simulink model "Aearial_Inspection_UAV_Simulation"  (R2023a)
settings: Solver=daessc  StartTime=0.0  StopTime=tf  MaxStep=0.1  MinStep=1e-30  RelTol=1e-4
values from neighbouring files (symbols this model uses):
  arm_start = 0    [InitScript.m]
  X = T*[x0;y0]    [line2circle.m]
undefined symbols (not defined in the file or in its folder): arm_end, DiscIntNeverNeededParam, F, is_gust_active, Light, MIL, Mode, Motor_data, params, Robotic_Arm_ASM_DataFile, Sensor_err, servo_specs, simple_env, stepper, Tm, wind_speed, xStack1, xStack2, Y, Z
libraries: sm_lib x399, nesl_utility x78, simulink x25, dspsrcs4 x16, simulink_extras x8, sharedtransform x7, aerolibwind2 x2, sharedutil x1
(part 1 of 12)
settings Model: Creator=mojta  LastModifiedBy=mojtaba
settings SolverCC: ZeroCrossControl=DisableAll
settings DebuggingCC: MaxConsecutiveZCsMsg=none  MaskedZcDiagnostic=none  IgnoredZcDiagnostic=none  UnconnectedInputMsg=warning  UnconnectedOutputMsg=warning  UnconnectedLineMsg=warning
settings ModelReferenceCC: EnableRefExpFcnMdlSchedulingChecks=on
settings RTWCC: DLArmComputeVersion=19.05
settings DiagnosticsConfigSet: SimMechanicsInvalidVisualProperty=none  SimMechanicsCrossSectionNullEdge=none  SimMechanicsRigidlyBoundBlock=none  SimMechanicsUnsatisfiedHighPriorityTargets=none

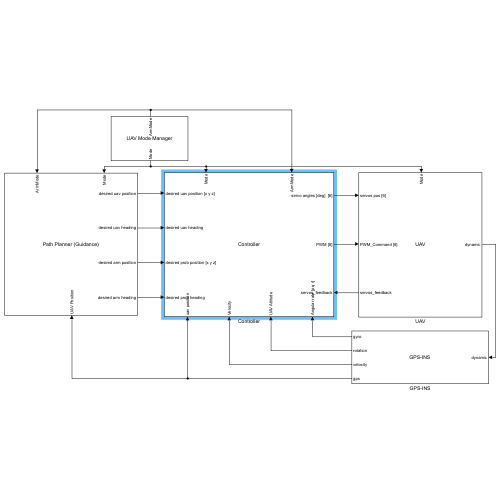
[thumbnail: Simulink's stored preview of the top-level diagram]
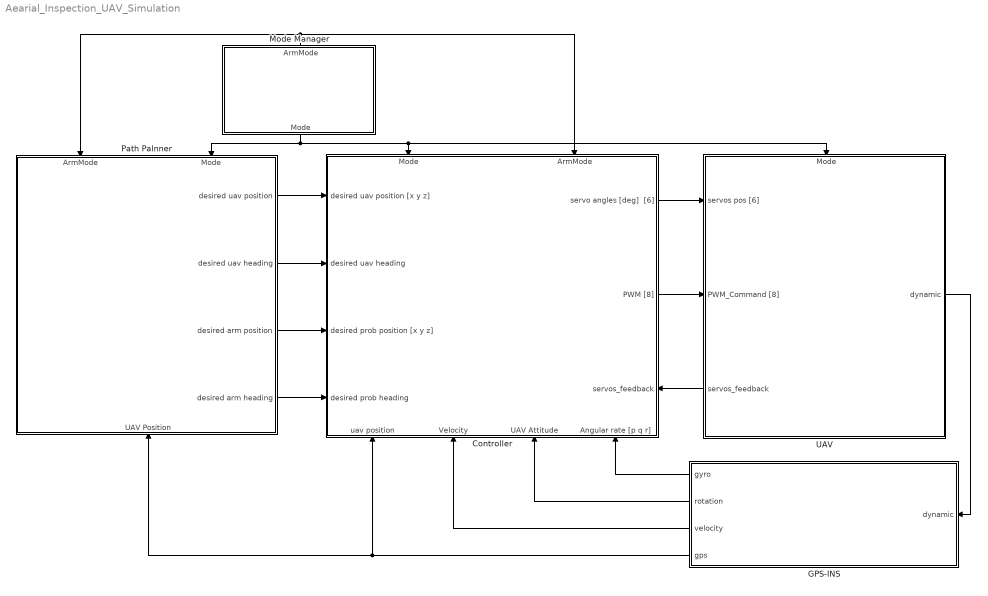
== system Aearial_Inspection_UAV_Simulation ==
  Controller : Subsystem
      settings: PortSchema="{\"entries\":[{\"content\":{\"sides\":[{\"content\":{\"connectorIds\":[\"In1\",\"In2\",\"In3\",\"In4\"]},\"type\":\"ConnectorPlacement.EquallySpacedRectSide\",\"uuid\":\"8cd7dc0d-1ffe-404b-8963-ef178fa92e53\"},{\"content\":{\"connectorIds\":[\"Out1\",\"Out2\",\"In11\"],\"side\":\"RIGHT\"},\"type\":\"ConnectorPlacement.EquallySpacedRectSide\",\"uuid\":\"919e0896-43af-402c-8143-9d4be52422e2\"},{\"content\":{\"connectorIds\":[\"In5\",\"In6\"],\"side\":\"TOP\"},\"type\":\"ConnectorPlacement.EquallySpacedRectSide\",\"uuid\":\"8ba6d734-f5ce-449a-9fca-978ebb325dd5\"},{\"content\":{\"connectorIds\":[\"In7\",\"In8\",\"In9\",\"In10\"],\"side\":\"BOTTOM\"},\"type\":\"ConnectorPlacement.EquallySpacedRectSide\",\"uuid\":\"341a769c-6dc0-48cd-a2a1-c1e2b0790a55\"}]},\"type\":\"ConnectorPlacement.EquallySpacedConnector\",\"uuid\":\"44d8020b-63e9-4f33-a120-ebcdce44349b\"}],\"packageUris\":[\"http://schema.mathworks.com/mf0/Connector/R2020b\"],\"version\":\"1.0\"}"
      mask Display: disp("Controller")
  GPS-INS : Subsystem
      mask Display: disp("GPS-INS")
  Mode Manager : Subsystem
      settings: PortSchema="{\"entries\":[{\"content\":{\"sides\":[{\"content\":{\"connectorIds\":[]},\"type\":\"ConnectorPlacement.EquallySpacedRectSide\",\"uuid\":\"ec3a6880-5567-4991-bb36-5b29953083f3\"},{\"content\":{\"connectorIds\":[],\"side\":\"RIGHT\"},\"type\":\"ConnectorPlacement.EquallySpacedRectSide\",\"uuid\":\"14318ee4-cc5e-4862-93f9-df06206ade9b\"},{\"content\":{\"connectorIds\":[\"Out2\"],\"side\":\"TOP\"},\"type\":\"ConnectorPlacement.EquallySpacedRectSide\",\"uuid\":\"762206d4-62cf-4133-8d53-9df821ce7e2e\"},{\"content\":{\"connectorIds\":[\"Out1\"],\"side\":\"BOTTOM\"},\"type\":\"ConnectorPlacement.EquallySpacedRectSide\",\"uuid\":\"6ead698c-d941-4f89-8f8b-414954de099a\"}]},\"type\":\"ConnectorPlacement.EquallySpacedConnector\",\"uuid\":\"33a2902f-a2fb-4f7e-8949-163cea2e732b\"}],\"packageUris\":[\"http://schema.mathworks.com/mf0/Connector/R2020b\"],\"version\":\"1.0\"}"
      mask Display: disp("UAV Mode Manager")
  Path Palnner : Subsystem
      settings: PortSchema="{\"entries\":[{\"content\":{\"sides\":[{\"content\":{\"connectorIds\":[]},\"type\":\"ConnectorPlacement.EquallySpacedRectSide\",\"uuid\":\"cb7ac4db-aadb-4fa9-9def-50252c1063a6\"},{\"content\":{\"connectorIds\":[\"Out1\",\"Out2\",\"Out3\",\"Out4\"],\"side\":\"RIGHT\"},\"type\":\"ConnectorPlacement.EquallySpacedRectSide\",\"uuid\":\"a421e774-a0ba-45ee-9144-209b429c5514\"},{\"content\":{\"connectorIds\":[\"In1\",\"In2\"],\"side\":\"TOP\"},\"type\":\"ConnectorPlacement.EquallySpacedRectSide\",\"uuid\":\"c25a837e-9178-40bf-ab38-1ae27b57d077\"},{\"content\":{\"connectorIds\":[\"In3\"],\"side\":\"BOTTOM\"},\"type\":\"ConnectorPlacement.EquallySpacedRectSide\",\"uuid\":\"24b9e0e9-1a2f-43ee-9fbc-f01c4afdd7a1\"}]},\"type\":\"ConnectorPlacement.EquallySpacedConnector\",\"uuid\":\"84baf3da-c25a-43bc-ab40-c057e0230948\"}],\"packageUris\":[\"http://schema.mathworks.com/mf0/Connector/R2020b\"],\"version\":\"1.0\"}"
      mask Display: disp("Path Planner (Guidance)")
  UAV : Subsystem
      mask init:
      | smiData = Aerial_Inspection_Octa_Rotor_DataFile();
      settings: PortSchema="{\"entries\":[{\"content\":{\"sides\":[{\"content\":{\"connectorIds\":[\"In1\",\"In2\",\"Out2\"]},\"type\":\"ConnectorPlacement.EquallySpacedRectSide\",\"uuid\":\"34cc31d8-8814-4b19-86b3-8c8699fa0f58\"},{\"content\":{\"connectorIds\":[\"Out1\"],\"side\":\"RIGHT\"},\"type\":\"ConnectorPlacement.EquallySpacedRectSide\",\"uuid\":\"29abd3e3-b5bd-4578-8682-c2c7537bb156\"},{\"content\":{\"connectorIds\":[\"In3\"],\"side\":\"TOP\"},\"type\":\"ConnectorPlacement.EquallySpacedRectSide\",\"uuid\":\"5d6ec585-4a55-4272-9af8-d672968573e8\"}]},\"type\":\"ConnectorPlacement.EquallySpacedConnector\",\"uuid\":\"91ac0284-653c-4c8b-a3f9-a6bca447147a\"}],\"packageUris\":[\"http://schema.mathworks.com/mf0/Connector/R2020b\"],\"version\":\"1.0\"}"
      mask Display: disp("UAV")
  wires:
  Mode Manager/1(Mode) -> Path Palnner/2(Mode), UAV/3(Mode), Controller/5(Mode)
  Path Palnner/1(desired uav position) -> Controller/1(desired uav position [x y z])
  Path Palnner/2(desired uav heading) -> Controller/2(desired uav heading)
  Path Palnner/3(desired arm position) -> Controller/3(desired prob position [x y z])
  Path Palnner/4(desired arm heading) -> Controller/4(desired prob heading)
  UAV/1(dynamic) -> GPS-INS/1(dynamic)
  GPS-INS/4(gps) -> Path Palnner/3(UAV Position), Controller/7(uav position)
  GPS-INS/3(velocity) -> Controller/8(Velocity)
  GPS-INS/2(rotation) -> Controller/9(UAV Attitude)
  GPS-INS/1("gyro ") -> Controller/10(Angular rate [p q r])
  Controller/1(servo angles [deg]  [6]) -> UAV/1(servos pos [6])
  Controller/2(PWM [8]) -> UAV/2(PWM_Command [8])
  Mode Manager/2(ArmMode) -> Path Palnner/1(ArmMode), Controller/6(ArmMode)
  UAV/2(servos_feedback) -> Controller/11(servos_feedback)

== system Aearial_Inspection_UAV_Simulation/Controller ==
  desired uav position [x y z] : Inport
  desired uav heading : Inport  Port=2
  desired prob position [x y z] : Inport  Port=3
  desired prob heading : Inport  Port=4
  Mode : Inport  Port=5
  ArmMode : Inport  Port=6
  uav position : Inport  Port=7
  Velocity : Inport  Port=8
  UAV Attitude : Inport  Port=9
  Angular rate [p q r] : Inport  Port=10
  servos_feedback : Inport  Port=11
  Arm Controller : Subsystem
      mask Display: disp("Arm Controller")
  Mixer : Subsystem
      mask init:
      | temp = Excel_Data;
      | 
      | Kt  = temp.K_T(1);
      | Km = temp.K_M(1);
      | r     = temp.d_motor;
      | 
      | K_ESC = zeros(8);
      | 
      | K_ESC(1,:)    = -Kt;
      | K_ESC(5:8,:) = [eye(4), -eye(4)];
      | 
      | for i=1:8
      | K_ESC(2,i) = -Kt*r(i,2);
      | K_ESC(3,i) = Kt*r(i,1);
      | K_ESC(4,i) = (-1)^(i)*Km;
      | end
      | 
      | inv_K_ESC = K_ESC^-1;
      | 
      | 
      | th = [0 0.5 0.55 0.6 0.65 0.75 0.85 1.]';
      | w = [0
      |     3703
      | 4005
      | 4289
      | 4575
      | 5091
      | 5635
      | 6374];
      | 
      | order = 3;
      | n = length(th);
      | A = zeros(n, order-1);
      | for i = 1 : n
      |     for j = 1:order
      |         A(i,j) = w(i)^j;
      |     end
      | end
      | 
      | a = (A'*A)^-1*A'*th;
      mask Display: disp("Mixer")
  To Workspace : ToWorkspace  VariableName=des_prob_pos  SaveFormat=Timeseries  SampleTime=-1
  UAV Controller : Subsystem
      mask init:
      | wc_Alt = 20;
      | 
      | wq = 200;
      | wp = wq;
      | wr = 50;
      | 
      | wc_x = 2;
      mask Display: disp("UAV Controller")
  servo angles [deg]  [6] : Outport
  PWM [8] : Outport  Port=2
  wires:
  UAV Controller/1(Controller Output [4]) -> Mixer/1(Controller output [4])
  desired prob position [x y z]/1 -> Arm Controller/1(desired prob pos [x,y,z]), To Workspace/1
  desired prob heading/1 -> Arm Controller/2(desired prob orientation)
  Mixer/1(PWM [8*1]) -> PWM [8]/1
  Arm Controller/1(servos pos [6]) -> servo angles [deg]  [6]/1
  desired uav position [x y z]/1 -> UAV Controller/1("desired position [xd, yd, zd]")
  desired uav heading/1 -> UAV Controller/2(desired Heading [psi_d])
  UAV Attitude/1 -> UAV Controller/5("Attitude (Euler Angles) [phi, theta, psi]"), Arm Controller/4(UAV Attitude)
  Angular rate [p q r]/1 -> UAV Controller/4(Angular Rate [p,q,r])
  uav position/1 -> UAV Controller/3(Position)
  Velocity/1 -> UAV Controller/6(Velocity)
  ArmMode/1 -> Arm Controller/5(ArmMode)
  Mode/1 -> Arm Controller/3(Mode)
  servos_feedback/1 -> Arm Controller/6(servos_feedback)

== system Aearial_Inspection_UAV_Simulation/GPS-INS ==
  dynamic : Inport
  GPS : Subsystem
  IMU : Subsystem
  Terminator : Terminator
  Terminator1 : Terminator
  Terminator2 : Terminator
  demux : Subsystem
  "gyro " : Outport
  rotation : Outport  Port=2
  velocity : Outport  Port=3
  gps : Outport  Port=4
  wires:
  dynamic/1 -> demux/1(Sensors)
  demux/5(Position) -> GPS/1(real Position data)
  IMU/1("gyro ") -> "gyro "/1
  IMU/4(rotation) -> rotation/1
  IMU/5(velocity IMU) -> velocity/1
  GPS/1("gps ") -> gps/1
  IMU/2(acc) -> Terminator/1
  IMU/3(mag) -> Terminator1/1
  GPS/2(gps velocity) -> Terminator2/1
  demux/1(Angular Velocity) -> IMU/1(real gyro data)
  demux/2(Quaternion) -> IMU/2(quaternions)
  demux/3(Acceleration) -> IMU/3(real acc data)
  demux/4(Velocity) -> IMU/4(real vel data)

== system Aearial_Inspection_UAV_Simulation/Mode Manager ==
  AND : Logic  IconShape=distinctive  AllPortsSameDT=off  OutDataTypeStr=boolean
  Cast To Double : DataTypeConversion  OutDataTypeStr=double  SaturateOnIntegerOverflow=off  RndMeth=Floor
  Clock : Clock
  Compare To Constant : simulink/Logic and Bit Operations/Compare To Constant  relop=>=  const=arm_start  OutDataTypeStr=boolean  ZeroCross=off
  Compare To Constant1 : simulink/Logic and Bit Operations/Compare To Constant  relop=<=  const=arm_end  OutDataTypeStr=boolean  ZeroCross=off
  Constant : Constant  Value=Mode
  Mode : Outport
  ArmMode : Outport  Port=2
  wires:
  Constant/1 -> Mode/1
  Cast To Double/1 -> ArmMode/1
  Clock/1 -> Compare To Constant1/1, Compare To Constant/1
  Compare To Constant/1 -> AND/1
  Compare To Constant1/1 -> AND/2
  AND/1 -> Cast To Double/1

== system Aearial_Inspection_UAV_Simulation/Path Palnner ==
  ArmMode : Inport
  Mode : Inport  Port=2
  UAV Position : Inport  Port=3
  Arm Guid : Subsystem
      mask Display: disp("Arm Planner")
  To Workspace : ToWorkspace  VariableName=des_pos  SaveFormat=Timeseries  SampleTime=-1
  To Workspace1 : ToWorkspace  VariableName=des_psi  SaveFormat=Timeseries  SampleTime=-1
  To Workspace2 : ToWorkspace  VariableName=des_arm_pos  SaveFormat=Timeseries  SampleTime=-1
  To Workspace3 : ToWorkspace  VariableName=des_arm_heading  SaveFormat=Timeseries  SampleTime=-1
  UAV_Guid : Subsystem
      mask Display: disp("UAV Guidance")
  desired uav position : Outport
  desired uav heading : Outport  Port=2
  desired arm position : Outport  Port=3
  desired arm heading : Outport  Port=4
  wires:
  Mode/1 -> Arm Guid/1(Mode), UAV_Guid/1(Mode)
  UAV Position/1 -> Arm Guid/3(uav_pos)
  UAV_Guid/1(desired_pos) -> To Workspace/1, desired uav position/1
  UAV_Guid/2(desired Heading) -> To Workspace1/1, desired uav heading/1
  Arm Guid/2(Arm Desired Orientation) -> To Workspace3/1, desired arm heading/1
  Arm Guid/1(Arm_desired_pos) -> To Workspace2/1, desired arm position/1
  ArmMode/1 -> Arm Guid/2(ArmMode)

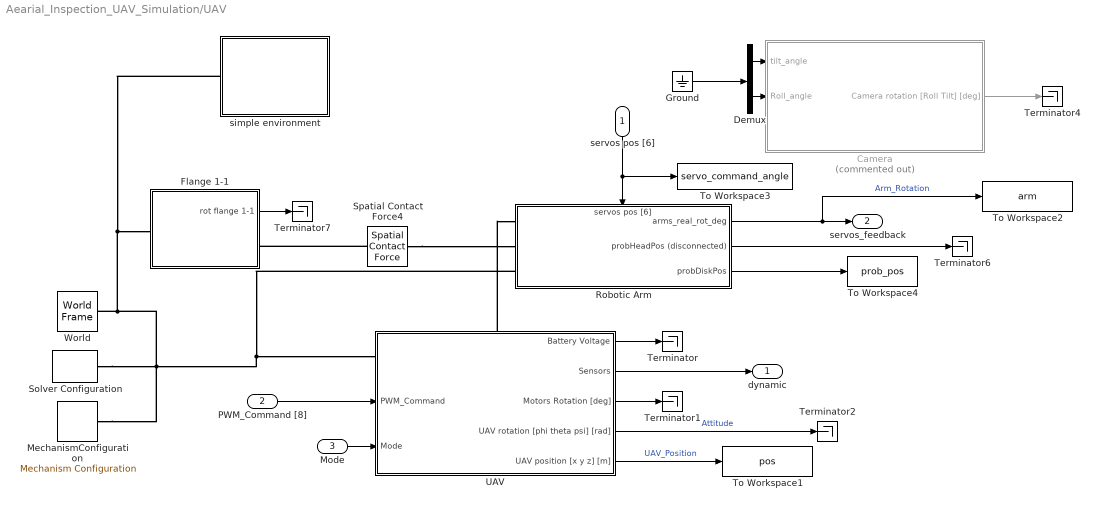
== system Aearial_Inspection_UAV_Simulation/UAV ==
  servos pos [6] : Inport  PortDimensions=6
  PWM_Command [8] : Inport  Port=2  PortDimensions=8
  Mode : Inport  Port=3
  Camera : Subsystem  Commented=on
      settings: MinAlgLoopOccurrences=on
      mask Display: image('D:\MS_Control_Project\pictures\CH3\Camera.JPG'); % Use "Edit Image" on toolstrip to change.
  Demux : Demux  Outputs=2
  Flange 1-1 : Subsystem
      mask init:
      | smiData = Flange_gate_DataFile();
      settings: MinAlgLoopOccurrences=on
  Ground : Ground
  MechanismConfiguration : sm_lib/Utilities/Mechanism Configuration  UniformGravity=Constant  GravityVector=[0 0 9.81]  GravityVectorUnits=m/s^2  LinearizationDelta=0.001  JointModeTransitionNonlinearIterations=2
  Robotic Arm : Subsystem  mask{smiData=Robotic_Arm_ASM_DataFile(), I_a0=20, I_a1=20, I_a2=20, I_w1=0.5, I_w2=0.5, I_w3=0.2, a0_maxTorque=200, a1_maxTorque=500, a2_maxTorque=200, w1_maxTorque=50, w2_maxTorque=50, w3_maxTorque=50, a0_maxVel=1, a1_maxVel=1, a2_maxVel=1, w1_maxVel=3, w2_maxVel=3, w3_maxVel=3}
      mask prompts: smiData "smData"; I_a0 "Servo a0"; I_a1 "Servo a1"; I_a2 "Servo a2"; I_w1 "Servo w1"; I_w2 "Servo w2"; I_w3 "Servo w3"; a0_maxTorque "Servo a0"; a1_maxTorque "Servo a1"; a2_maxTorque "Servo a2"; w1_maxTorque "Servo w1"; w2_maxTorque "Servo w2"; w3_maxTorque "Servo w3"; a0_maxVel "Servo a0"; a1_maxVel "Servo a1"; a2_maxVel "Servo a2"; w1_maxVel "Servo w1"; w2_maxVel "Servo w2"; w3_maxVel "Servo w3"
      mask init:
      | main
      settings: PortSchema="{\"entries\":[{\"content\":{\"sides\":[{\"content\":{\"connectorIds\":[\"LConn1\",\"LConn2\",\"LConn3\"]},\"type\":\"ConnectorPlacement.EquallySpacedRectSide\",\"uuid\":\"03f1ddf6-71cc-47f6-8398-5c3f516e61c7\"},{\"content\":{\"connectorIds\":[\"Out1\",\"Out2\",\"Out3\"],\"side\":\"RIGHT\"},\"type\":\"ConnectorPlacement.EquallySpacedRectSide\",\"uuid\":\"d8ba576a-9aaa-4705-a901-8658d79ba4ef\"},{\"content\":{\"connectorIds\":[\"In1\"],\"side\":\"TOP\"},\"type\":\"ConnectorPlacement.EquallySpacedRectSide\",\"uuid\":\"02397d5d-c4e1-4539-9121-e7da8e23bc4c\"}]},\"type\":\"ConnectorPlacement.EquallySpacedConnector\",\"uuid\":\"067dd81b-c51f-4725-9db0-fb64c43a5cf5\"}],\"packageUris\":[\"http://schema.mathworks.com/mf0/Connector/R2020b\"],\"version\":\"1.0\"}"
      mask DialogControl ParameterGroupVar Prompt: Data
      mask DialogControl ParameterGroupVar_copy Prompt: Inertia on Servos
      mask DialogControl ParameterGroupVar_copy_copy Prompt: Max Torque of Servos
      mask DialogControl ParameterGroupVar_copy_copy_copy Prompt: Max Velocity of Servos
  Solver Configuration : nesl_utility/Solver Configuration  PhysicalDomain=network_engine_domain  SubClassName=solver  LeftPortType=input  RightPortType=generic  Tones=[]  Harmonics=[]  SimulateNoise=off  Profile=off  UseLocalSampling=off  EnableSwitchedLinearOptims=on  FrequencyDomain=off  UseCCode=off  RelTol=0.001  AbsTol=1e-06  MinStep=1e-09  ToWorkspace=off  RevertToSquareIcSolve=off  NumHomotopyIterations=100  PhasorMode=off  PhasorModeNumHarmonics=1  ConsistencySolver=NEWTON_FTOL  IndexReductionMethod=DerivativeReplacement  DoDC=off  ResidualTolerance=1e-09  ConsistencyTolSource=GLOBAL  ConsistencyAbsTol=0.001  ConsistencyRelTol=0.001  ConsistencyTolFactor=0.001  UseLocalSolver=off  LocalSolverChoice=NE_BACKWARD_EULER_ADVANCER  ResolveIndetEquations=on  FunctionEvalNumThread=1  LocalSolverSampleTime=0.001  DoFixedCost=off  MaxNonlinIter=3  MaxModeIter=2  ComputeImpulses=off  ImpulseIterations=2  LinearAlgebra=auto  LinearAlgebraNumThread=0  EquationFormulation=NE_TIME_EF  DelaysMemoryBudget=1024  AutomaticFiltering=on  FilteringTimeConstant=0.001  PartitionStorageMethod=AS_NEEDED  PartitionMemoryBudget=1024  PartitionMethod=ROBUST
  Spatial Contact Force4 : sm_lib/Forces and Torques/Spatial Contact Force  SenseContactBaseRotation=off  SenseContactBaseTranslation=off  CoefficientOfDynamicFriction=0.3  CoefficientOfStaticFriction=0.5  NormalDamping=1000  NormalDampingUnits=N/(m/s)  SenseContactSignal=off  NormalStiffness=1000  NormalStiffnessUnits=N/m  FrictionalCriticalVelocity=1e-3  FrictionalCriticalVelocityUnits=m/s  ZeroCrossDetectContactStartAndEnd=off  SenseContactFollowerRotation=off  SenseContactFollowerTranslation=off  FrictionType=SmoothStickSlip  SenseFrictionalForceMagnitude=off  SenseNormalForceMagnitude=off  NormalForceType=SmoothSpringDamper  SenseNormalVelocity=off  SenseSeparationDistance=off  SenseTangentialVelocity=off  NormalTransitionRegionWidth=1e-3  NormalTransitionRegionWidthUnits=m
  Terminator{,1..2,4,6..7} (6 alike) : Terminator
  To Workspace1 : ToWorkspace  VariableName=pos  SaveFormat=Timeseries  SampleTime=-1
  To Workspace2 : ToWorkspace  VariableName=arm  SaveFormat=Timeseries  SampleTime=-1
  To Workspace3 : ToWorkspace  VariableName=servo_command_angle  SaveFormat=Timeseries  SampleTime=-1
  To Workspace4 : ToWorkspace  VariableName=prob_pos  SaveFormat=Timeseries  SampleTime=-1
  UAV : Subsystem
      settings: MinAlgLoopOccurrences=on  PortSchema="{\"entries\":[{\"content\":{\"sides\":[{\"content\":{\"connectorIds\":[\"LConn1\",\"In1\",\"In2\"]},\"type\":\"ConnectorPlacement.EquallySpacedRectSide\",\"uuid\":\"3a522cf1-0d2e-42a1-8abc-fdb0da215095\"},{\"content\":{\"connectorIds\":[\"Out1\",\"Out2\",\"Out3\",\"Out4\",\"Out5\"],\"side\":\"RIGHT\"},\"type\":\"ConnectorPlacement.EquallySpacedRectSide\",\"uuid\":\"0b06edfd-f156-4bc5-9eca-7fe97f182038\"},{\"content\":{\"connectorIds\":[\"LConn2\"],\"side\":\"TOP\"},\"type\":\"ConnectorPlacement.EquallySpacedRectSide\",\"uuid\":\"5d149f1b-6095-4c3b-bbee-46e9e9cd7497\"}]},\"type\":\"ConnectorPlacement.EquallySpacedConnector\",\"uuid\":\"072866d9-af86-4096-8e43-cca5dedb3158\"}],\"packageUris\":[\"http://schema.mathworks.com/mf0/Connector/R2020b\"],\"version\":\"1.0\"}"
      mask Display: image('D:\MS_Control_Project\pictures\CH5\UAV.JPG'); % Use "Edit Image" on toolstrip to change.
  World : sm_lib/Frames and Transforms/World Frame
  simple environment : Subsystem
  dynamic : Outport
  servos_feedback : Outport  Port=2
  wires:
  Demux/1 -> Camera/1(tilt_angle)
  PWM_Command [8]/1 -> UAV/1(PWM_Command)
  Robotic Arm/3(probDiskPos) -> To Workspace4/1
  UAV/1(Battery Voltage) -> Terminator/1
  UAV/2(Sensors) -> dynamic/1
  servos pos [6]/1 -> To Workspace3/1, Robotic Arm/1(servos pos [6])
  Flange 1-1/1(rot flange 1-1) -> Terminator7/1
  Robotic Arm/1(arms_real_rot_deg) -> servos_feedback/1, To Workspace2/1  "Arm_Rotation"
  Demux/2 -> Camera/2(Roll_angle)
  UAV/4(UAV rotation [phi theta psi] [rad]) -> Terminator2/1  "Attitude"
  Ground/1 -> Demux/1
  Camera/1(Camera rotation [Roll Tilt] [deg]) -> Terminator4/1
  UAV/3(Motors Rotation [deg]) -> Terminator1/1
  UAV/5(UAV position [x y z] [m]) -> To Workspace1/1  "UAV_Position"
  Robotic Arm/2(probHeadPos (disconnected)) -> Terminator6/1
  Mode/1 -> UAV/2(Mode)
  connections:
  MechanismConfiguration/RConn1 -- Solver Configuration/RConn1 -- simple environment/LConn1 -- Flange 1-1/LConn1 -- World/RConn1 -- Robotic Arm/LConn3 -- UAV/LConn1
  UAV/LConn2 -- Robotic Arm/LConn1
  Spatial Contact Force4/LConn1 -- Flange 1-1/RConn1
  Spatial Contact Force4/RConn1 -- Robotic Arm/LConn2

== system Aearial_Inspection_UAV_Simulation/Controller/Arm Controller ==
  desired prob pos [x,y,z] : Inport
  desired prob orientation : Inport  Port=2  PortDimensions=1
  Mode : Inport  Port=3
  UAV Attitude : Inport  Port=4  PortDimensions=3
  ArmMode : Inport  Port=5
  servos_feedback : Inport  Port=6
  Arm and Wrist Inv-kinematics : Subsystem
  Compare To Constant : simulink/Logic and Bit Operations/Compare To Constant  relop===  const=2  OutDataTypeStr=boolean
  Compare To Constant1 : simulink/Logic and Bit Operations/Compare To Constant  relop===  const=5  OutDataTypeStr=boolean
  Compare To Constant2 : simulink/Logic and Bit Operations/Compare To Constant  relop===  const=2  OutDataTypeStr=boolean
  Compare To Constant3 : simulink/Logic and Bit Operations/Compare To Constant  relop===  const=5  OutDataTypeStr=boolean
  Enabled Subsystem : Subsystem  TreatAsAtomicUnit=on
  NOT : Logic  Operator=NOT  IconShape=distinctive  AllPortsSameDT=off  OutDataTypeStr=boolean
  OR : Logic  Operator=OR  IconShape=distinctive  AllPortsSameDT=off  OutDataTypeStr=boolean
  Subsystem : Subsystem
  Sum : Sum  Inputs=++|
  Sum1 : Sum  Inputs=++|
  servos pos [6] : Outport
  wires:
  Compare To Constant1/1 -> Arm and Wrist Inv-kinematics/Enable
  Mode/1 -> Compare To Constant/1, Compare To Constant2/1, Compare To Constant3/1, Compare To Constant1/1, Arm and Wrist Inv-kinematics/1(Mode)
  Enabled Subsystem/1(Servo pos [6]) -> Sum1/1
  desired prob pos [x,y,z]/1 -> Arm and Wrist Inv-kinematics/2(desired prob pos [x,y,z])
  Compare To Constant/1 -> Enabled Subsystem/Enable
  desired prob orientation/1 -> Arm and Wrist Inv-kinematics/3(desired prob orientation)
  Arm and Wrist Inv-kinematics/1(servos pos [6]) -> Sum/2
  Sum/1 -> servos pos [6]/1
  UAV Attitude/1 -> Arm and Wrist Inv-kinematics/4(UAV Attitude)
  ArmMode/1 -> Arm and Wrist Inv-kinematics/5(ArmMode)
  servos_feedback/1 -> Arm and Wrist Inv-kinematics/6(servos_feedback)
  Compare To Constant2/1 -> OR/1
  Compare To Constant3/1 -> OR/2
  OR/1 -> NOT/1
  Sum1/1 -> Sum/1
  Subsystem/1(Out1) -> Sum1/2
  NOT/1 -> Subsystem/1(In1)

== system Aearial_Inspection_UAV_Simulation/Controller/Mixer ==
  Controller output [4] : Inport  PortDimensions=4
  Constant : Constant  Value=zeros(4,1)
  Constant1 : Constant  Value=3
  Gain : Gain  Gain=inv_K_ESC  Multiplication=Matrix(K*u)
  Gain1 : Gain  Gain=a(3)
  Gain2 : Gain  Gain=a(2)
  Gain3 : Gain  Gain=a(1)
  Mux : Mux  Inputs=2
  N 2 gr : Gain  Gain=[1000/9.81*[1 1 1] 1]
  Power : Math  Operator=square
  Power1 : Math  Operator=pow
  Saturation : Saturate  UpperLimit=(6374*2*pi/60)^2  LowerLimit=0  ZeroCross=off
  Saturation1 : Saturate  UpperLimit=1  LowerLimit=0  ZeroCross=off
  Scope : Scope
  Scope1 : Scope
  Scope2 : Scope
  Sqrt : Sqrt
  Sum : Sum  Inputs=3
  rad/s to RPM : Gain  Gain=60/2/pi
  PWM [8*1] : Outport
  wires:
  N 2 gr/1 -> Mux/1
  Saturation1/1 -> Scope/1, PWM [8*1]/1
  Gain1/1 -> Sum/1
  Gain3/1 -> Sum/3
  Controller output [4]/1 -> Scope1/1, N 2 gr/1
  Saturation/1 -> Sqrt/1
  rad/s to RPM/1 -> Scope2/1, Gain3/1, Power1/1, Power/1
  Gain2/1 -> Sum/2
  Sqrt/1 -> rad/s to RPM/1
  Power/1 -> Gain2/1
  Sum/1 -> Saturation1/1
  Constant/1 -> Mux/2
  Power1/1 -> Gain1/1
  Constant1/1 -> Power1/2
  Mux/1 -> Gain/1
  Gain/1 -> Saturation/1

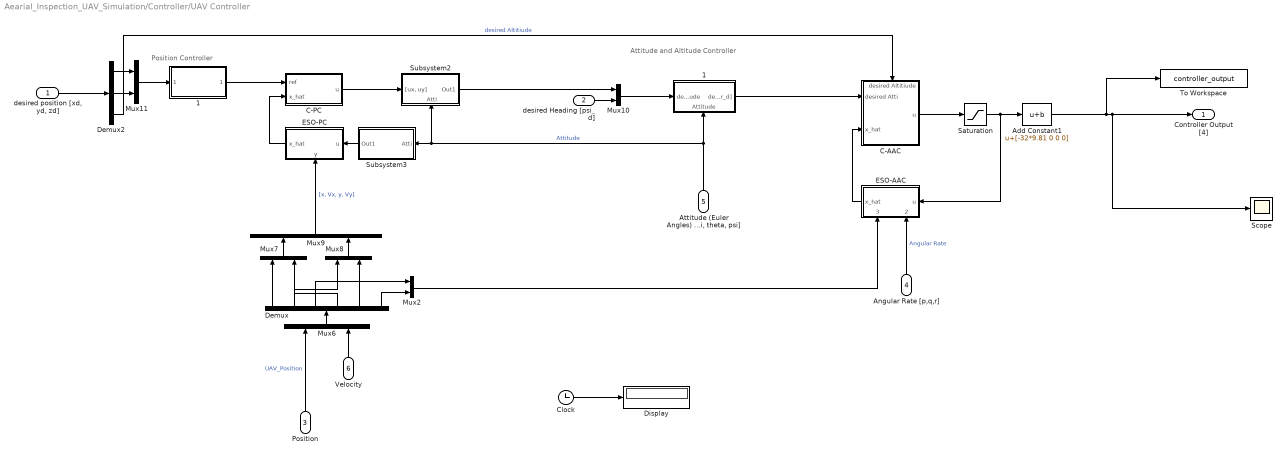
== system Aearial_Inspection_UAV_Simulation/Controller/UAV Controller ==
  note: Attitude and Altitude Controller
  note: Position Controller
  "desired position [xd, yd, zd]" : Inport  PortDimensions=3
  desired Heading [psi_d] : Inport  Port=2  PortDimensions=1
  Position : Inport  Port=3  PortDimensions=3
  Angular Rate [p,q,r] : Inport  Port=4  PortDimensions=3
  "Attitude (Euler Angles) [phi, theta, psi]" : Inport  Port=5  PortDimensions=3
  Velocity : Inport  Port=6  PortDimensions=3
  "      1" : Subsystem  mask{ff_on=0, wphi=wp/4, wpsi=wr/4}
      mask prompts: ff_on "is Feed Forward Enable"; wphi "phi and theta Channel freq"; wpsi "psi Channel freq"
      mask init:
      | K = [wphi 0 0;0 wphi 0;0 0 wpsi];
      | C = [0 ff_on      0 0      0 0
      |      0 0      0 ff_on      0 0
      |      0 0      0 0      0 ff_on];
      settings: PortSchema="{\"entries\":[{\"content\":{\"sides\":[{\"content\":{\"connectorIds\":[\"In1\"]},\"type\":\"ConnectorPlacement.EquallySpacedRectSide\",\"uuid\":\"d7bfb74f-f0ef-45e8-b402-84c976e030ff\"},{\"content\":{\"connectorIds\":[\"Out1\"],\"side\":\"RIGHT\"},\"type\":\"ConnectorPlacement.EquallySpacedRectSide\",\"uuid\":\"7a56635f-9db1-4285-a1b6-a2387fe77a8c\"},{\"content\":{\"connectorIds\":[],\"side\":\"TOP\"},\"type\":\"ConnectorPlacement.EquallySpacedRectSide\",\"uuid\":\"8927570d-ca43-4684-a275-ba6cf3010bd2\"},{\"content\":{\"connectorIds\":[\"In2\"],\"side\":\"BOTTOM\"},\"type\":\"ConnectorPlacement.EquallySpacedRectSide\",\"uuid\":\"c03033a2-2d15-4ba6-80ad-a3592136c9e5\"}]},\"type\":\"ConnectorPlacement.EquallySpacedConnector\",\"uuid\":\"5c6a6a0d-05db-4861-9314-e27434e60dad\"}],\"packageUris\":[\"http://schema.mathworks.com/mf0/Connector/R2020b\"],\"version\":\"1.0\"}"
      mask Display: disp("EU2BAR")
  "     1" : Subsystem  mask{wx=50, wy=50}
      mask init:
      | Bx = zeros(3,1);
      | Bx(end) = wx^3;
      | 
      | Ax = zeros(3);
      | Ax(1,2) = 1;
      | Ax(2,3) = 1;
      | Ax(end,:) = [-wx^3 -3*wx^2 -3*wx];
      | 
      | By = zeros(3,1);
      | By(end) = wy^3;
      | 
      | Ay = zeros(3);
      | Ay(1,2) = 1;
      | Ay(2,3) = 1;
      | Ay(end,:) = [-wy^3 -3*wy^2 -3*wy];
      mask Display: disp("TD-PC")
  Add Constant1 : Bias  Bias=[-32*9.81 0 0 0]  SaturateOnIntegerOverflow=off
  "C-AAC " : Subsystem
      settings: PortSchema="{\"entries\":[{\"content\":{\"sides\":[{\"content\":{\"connectorIds\":[\"In1\",\"In2\"]},\"type\":\"ConnectorPlacement.EquallySpacedRectSide\",\"uuid\":\"0074a7af-5369-4567-a570-5214c890c1e4\"},{\"content\":{\"connectorIds\":[\"Out1\"],\"side\":\"RIGHT\"},\"type\":\"ConnectorPlacement.EquallySpacedRectSide\",\"uuid\":\"74f23e42-f7b0-4104-8eab-960110f0734e\"},{\"content\":{\"connectorIds\":[\"In3\"],\"side\":\"TOP\"},\"type\":\"ConnectorPlacement.EquallySpacedRectSide\",\"uuid\":\"3809b58d-5d28-4fa1-bb5c-40abfdb463ef\"}]},\"type\":\"ConnectorPlacement.EquallySpacedConnector\",\"uuid\":\"2144d4c9-afd4-4ceb-a08a-cb907e035127\"}],\"packageUris\":[\"http://schema.mathworks.com/mf0/Connector/R2020b\"],\"version\":\"1.0\"}"
  C-PC : Subsystem
  Clock : Clock
  Demux : Demux  Outputs=6
  Demux2 : Demux  Outputs=3
  Display : Display
  ESO-AAC : Subsystem  mask{w_z=wc_Alt/2, w_p=wp/2, w_q=wq/2, w_r=wr/2, zeta=1}
      mask prompts: w_z "Alt Channel freq"; w_p "roll Channel freq"; w_q "pitch Channel freq"; w_r "yaw Channel freq"; zeta "damping coef"
      mask init:
      | C = [eye(5) zeros(5,4)];
      | 
      | params = Excel_Data;
      | m = params.M;
      | I = params.I;
      | 
      | Ix = I(1,1);
      | Iy = I(2,2);
      | Iz = I(3,3);
      | Ixz = I(1,3);
      | 
      | B = [0 0 0 0;1/m 0 0 0;0 Iz/(Iz*Ix-Ixz^2) 0 -Ixz/(Iz*Ix-Ixz^2);
      |      0 0 1/Iy 0;0 -Ixz/(Iz*Ix-Ixz^2) 0 Ix/(Iz*Ix-Ixz^2);zeros(4)];
      | 
      | L1 = 3*w_z;
      | L2 = 3*w_z^2;
      | L7 = m*w_z^3; 
      |  
      | L4 = 2*zeta*w_q;
      | L6 = (0.25*L4^2 + w_q^2*(1-zeta^2))/0.250549;
      | 
      | L3 = 2*zeta*w_p;
      | L5 = w_p^2*Ix;
      | 
      | L8 = 2*zeta*w_r;
      | L9 = w_r^2*Iz;
      | 
      | % syms L3 L5 L8 L9 L10 L11 a1 a2 a3 s wz wx real
      | 
      | A1 = [0 1 0 0 0;
      |     zeros(4,5)];
      | 
      | B1 = [0 0 0 0;1/m 0 0 0;zeros(3,1) I^-1];
      | A = [A1 B1
      |     zeros(4,9)];
      | 
      | 
      | L = [L1 0 0 0 0;L2 0 0 0 0;0 0 L3 0 0;0 0 0 L4 0;0 0 0 0 L8;L7 0 0 0 0;0 0 L5 0 0;
      |      0  0 0 L6 0; 0 0 0 0 L9];
      |  
      | eig(A-L*C)
      settings: PortSchema="{\"entries\":[{\"content\":{\"sides\":[{\"content\":{\"connectorIds\":[\"In1\"]},\"type\":\"ConnectorPlacement.EquallySpacedRectSide\",\"uuid\":\"d7bfb74f-f0ef-45e8-b402-84c976e030ff\"},{\"content\":{\"connectorIds\":[\"Out1\"],\"side\":\"RIGHT\"},\"type\":\"ConnectorPlacement.EquallySpacedRectSide\",\"uuid\":\"7a56635f-9db1-4285-a1b6-a2387fe77a8c\"},{\"content\":{\"connectorIds\":[],\"side\":\"TOP\"},\"type\":\"ConnectorPlacement.EquallySpacedRectSide\",\"uuid\":\"8927570d-ca43-4684-a275-ba6cf3010bd2\"},{\"content\":{\"connectorIds\":[\"In2\",\"In3\"],\"side\":\"BOTTOM\"},\"type\":\"ConnectorPlacement.EquallySpacedRectSide\",\"uuid\":\"f91df5b2-ed55-4d65-a094-b76377ad5e05\"}]},\"type\":\"ConnectorPlacement.EquallySpacedConnector\",\"uuid\":\"5c6a6a0d-05db-4861-9314-e27434e60dad\"}],\"packageUris\":[\"http://schema.mathworks.com/mf0/Connector/R2020b\"],\"version\":\"1.0\"}"
      mask Display: disp("ESO-AAC")
  ESO-PC : Subsystem  mask{w=wc_x}
      mask prompts: w "natural freq of complex pole"
      mask init:
      | L1 = 3*w;
      | L2 = 3*w^2;
      | L3 = w^3;
      | 
      | L4 = L1;
      | L5 = L2;
      | L6 = L3;
      | 
      | L = [L1 0 0 0;
      |      L2 0 0 0 
      |      0 0 L4 0
      |      0 0 L5 0
      |      L3 0 0 0
      |      0 0 L6 0];
      | 
      | A = [0 1 0 0
      |      0 0 0 0
      |      0 0 0 1
      |      0 0 0 0];
      | M = [0 0
      |     1 0
      |     0 0
      |     0 1];
      | C = [eye(4) zeros(4,2)];
      | 
      | A = [A M;zeros(2,6)];
      | 
      | B = [0 0;1 0;0 0;0 1;0 0;0 0];
      settings: PortSchema="{\"entries\":[{\"content\":{\"sides\":[{\"content\":{\"connectorIds\":[\"In1\"]},\"type\":\"ConnectorPlacement.EquallySpacedRectSide\",\"uuid\":\"d7bfb74f-f0ef-45e8-b402-84c976e030ff\"},{\"content\":{\"connectorIds\":[\"Out1\"],\"side\":\"RIGHT\"},\"type\":\"ConnectorPlacement.EquallySpacedRectSide\",\"uuid\":\"7a56635f-9db1-4285-a1b6-a2387fe77a8c\"},{\"content\":{\"connectorIds\":[],\"side\":\"TOP\"},\"type\":\"ConnectorPlacement.EquallySpacedRectSide\",\"uuid\":\"8927570d-ca43-4684-a275-ba6cf3010bd2\"},{\"content\":{\"connectorIds\":[\"In2\"],\"side\":\"BOTTOM\"},\"type\":\"ConnectorPlacement.EquallySpacedRectSide\",\"uuid\":\"2b6c045b-0b63-4552-873e-a472e925fa36\"}]},\"type\":\"ConnectorPlacement.EquallySpacedConnector\",\"uuid\":\"5c6a6a0d-05db-4861-9314-e27434e60dad\"}],\"packageUris\":[\"http://schema.mathworks.com/mf0/Connector/R2020b\"],\"version\":\"1.0\"}"
      mask Display: disp("ESO-PC")
  Mux{2,6..11} (7 alike) : Mux  Inputs=2
  Saturation : Saturate  UpperLimit=[150 100 100 1.8*4]  LowerLimit=[-150 -100 -100 -1.8*4]  ZeroCross=off
  Scope : Scope
  Subsystem2 : Subsystem
      settings: PortSchema="{\"entries\":[{\"content\":{\"sides\":[{\"content\":{\"connectorIds\":[\"In1\"]},\"type\":\"ConnectorPlacement.EquallySpacedRectSide\",\"uuid\":\"1f5be12c-0015-40b2-bce0-3a0d27346b90\"},{\"content\":{\"connectorIds\":[\"Out1\"],\"side\":\"RIGHT\"},\"type\":\"ConnectorPlacement.EquallySpacedRectSide\",\"uuid\":\"d291273e-1e98-4271-b999-541a78db916f\"},{\"content\":{\"connectorIds\":[],\"side\":\"TOP\"},\"type\":\"ConnectorPlacement.EquallySpacedRectSide\",\"uuid\":\"31981d06-c4a1-43d5-a7b9-a24549041434\"},{\"content\":{\"connectorIds\":[\"In2\"],\"side\":\"BOTTOM\"},\"type\":\"ConnectorPlacement.EquallySpacedRectSide\",\"uuid\":\"660fd505-562e-46c1-ac20-75e83f511c9b\"}]},\"type\":\"ConnectorPlacement.EquallySpacedConnector\",\"uuid\":\"1e4f524b-2827-4918-a88e-6164cba08db9\"}],\"packageUris\":[\"http://schema.mathworks.com/mf0/Connector/R2020b\"],\"version\":\"1.0\"}"
      mask Display: disp("Acc2Tilt")
  Subsystem3 : Subsystem
      mask Display: disp("Tilt2Acc")
  To Workspace : ToWorkspace  VariableName=controller_output  SaveFormat=Timeseries  SampleTime=-1
  Controller Output [4] : Outport  PortDimensions=4
  wires:
  Mux2/1 -> ESO-AAC/3("[Alt, Climb rate]")
  Angular Rate [p,q,r]/1 -> ESO-AAC/2(Angular Rate [p,q,r])  "Angular Rate"
  Demux2/3 -> "C-AAC "/3(desired Altitiude)  "desired Altitiude"
  Mux8/1 -> Mux9/2
  "     1"/1("[xd, xd_dot, xd_2dot] [yd, yd_dot, yd_2dot]") -> C-PC/1(ref)
  Mux6/1 -> Demux/1
  ESO-AAC/1(x_hat) -> "C-AAC "/2(x_hat)
  Position/1 -> Mux6/1  "UAV_Position"
  C-PC/1(u) -> Subsystem2/1("[ux, uy]")
  Add Constant1/1 -> To Workspace/1, Scope/1, Controller Output [4]/1
  Demux2/2 -> Mux11/2
  ESO-PC/1(x_hat) -> C-PC/2(x_hat)
  Subsystem2/1(Out1) -> Mux10/1
  "desired position [xd, yd, zd]"/1 -> Demux2/1
  Mux11/1 -> "     1"/1("[xd, yd]")
  Mux7/1 -> Mux9/1
  Demux2/1 -> Mux11/1
  Clock/1 -> Display/1
  Mux9/1 -> ESO-PC/2(y)  "[x, Vx, y, Vy]"
  Velocity/1 -> Mux6/2
  Demux/2 -> Mux8/1
  Subsystem3/1(Out1) -> ESO-PC/1(u)
  Saturation/1 -> Add Constant1/1, ESO-AAC/1(u)
  Demux/6 -> Mux2/2
  desired Heading [psi_d]/1 -> Mux10/2
  Demux/5 -> Mux8/2
  Mux10/1 -> "      1"/1(desired Attitude)
  "Attitude (Euler Angles) [phi, theta, psi]"/1 -> "      1"/2(Attitude), Subsystem3/1(Atti), Subsystem2/2(Atti)  "Attitude"
  "      1"/1("desired Angular rate [p_d, q_d, r_d]") -> "C-AAC "/1(desired Atti)
  "C-AAC "/1(u) -> Saturation/1
  Demux/3 -> Mux2/1
  Demux/1 -> Mux7/1
  Demux/4 -> Mux7/2

== system Aearial_Inspection_UAV_Simulation/GPS-INS/GPS ==
  real Position data : Inport  PortDimensions=3
  Gain : Gain  Commented=on  Gain=Sensor_err.gps.filt
  Integrator : Integrator  Commented=on
  Subsystem : Subsystem
  Sum : Sum  Commented=on  Inputs=+-
  Transport Delay : TransportDelay  DelayTime=0.001
  "gps " : Outport
  gps velocity : Outport  Port=2
  wires:
  Transport Delay/1 -> Subsystem/1(real Position data)
  Integrator/1 -> Sum/2
  Gain/1 -> Integrator/1, gps velocity/1
  Sum/1 -> Gain/1
  Subsystem/1(gps output) -> Sum/1, "gps "/1
  real Position data/1 -> Transport Delay/1

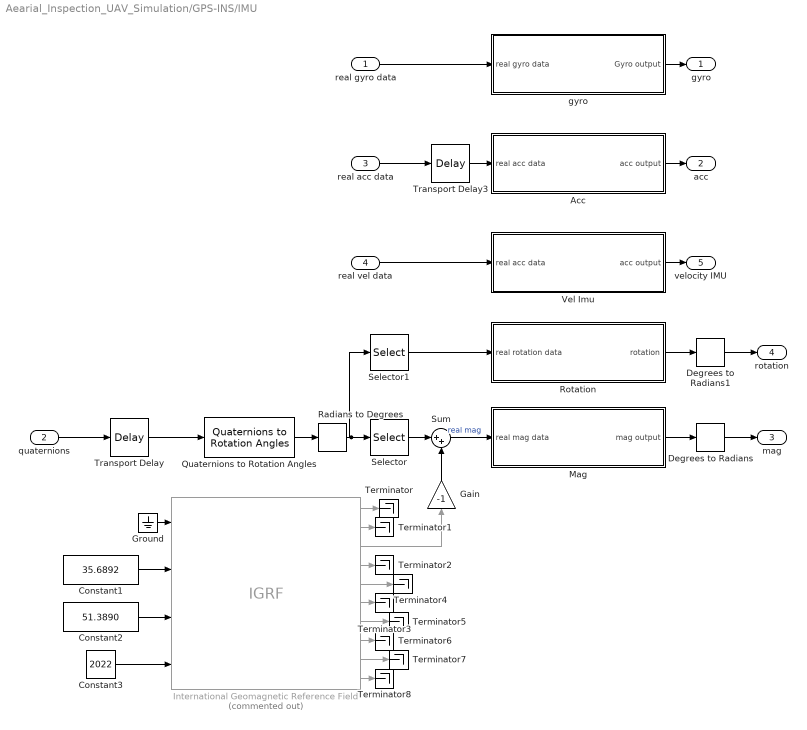
== system Aearial_Inspection_UAV_Simulation/GPS-INS/IMU ==
  real gyro data : Inport  PortDimensions=3
  quaternions : Inport  Port=2  PortDimensions=4
  real acc data : Inport  Port=3  PortDimensions=3
  real vel data : Inport  Port=4  PortDimensions=3
  Acc : Subsystem
  Constant1 : Constant  Value=35.6892
  Constant2 : Constant  Value=51.3890
  Constant3 : Constant  Value=2022
  Degrees to Radians : simulink_extras/Transformations/Degrees to Radians
  Degrees to Radians1 : simulink_extras/Transformations/Degrees to Radians
  Gain : Gain  Gain=-1
  Ground : Ground
  International Geomagnetic Reference Field : IGRF  Commented=on  month=January  day=1  year=2020
      settings: AttributesFormatString=%<generation>
  Mag : Subsystem
  Quaternions to Rotation Angles : sharedtransform/Quaternions to Rotation Angles  rotationOrder=ZYX  aMode=aMode
  Radians to Degrees : simulink_extras/Transformations/Radians to Degrees
  Rotation : Subsystem
  Selector : Selector  InputPortWidth=3  IndexOptions=Index vector (dialog)  Indices=1  OutputSizes=1
  Selector1 : Selector  InputPortWidth=3  IndexOptions=Index vector (dialog)  Indices=[3 2 1]  OutputSizes=1
  Sum : Sum  Inputs=|++
  Terminator{,1..8} (9 alike) : Terminator
  Transport Delay : TransportDelay  DelayTime=0.001  InitialOutput=[1 0 0 0]
  Transport Delay3 : TransportDelay  DelayTime=0.001
  Vel Imu : Subsystem
  gyro : Subsystem
  "gyro " : Outport
  acc : Outport  Port=2
  mag : Outport  Port=3
  rotation : Outport  Port=4
  velocity IMU : Outport  Port=5
  wires:
  Selector/1 -> Sum/1
  real acc data/1 -> Transport Delay3/1
  real vel data/1 -> Vel Imu/1(real acc data)
  International Geomagnetic Reference Field/9 -> Terminator7/1
  quaternions/1 -> Transport Delay/1
  Constant2/1 -> International Geomagnetic Reference Field/3
  International Geomagnetic Reference Field/5 -> Terminator4/1
  Ground/1 -> International Geomagnetic Reference Field/1
  Radians to Degrees/1 -> Selector1/1, Selector/1
  real gyro data/1 -> gyro/1(real gyro data)
  International Geomagnetic Reference Field/8 -> Terminator6/1
  Quaternions to Rotation Angles/1 -> Radians to Degrees/1
  Rotation/1(rotation) -> Degrees to Radians1/1
  Selector1/1 -> Rotation/1(real rotation data)
  International Geomagnetic Reference Field/7 -> Terminator5/1
  Degrees to Radians/1 -> mag/1
  Degrees to Radians1/1 -> rotation/1
  International Geomagnetic Reference Field/3 -> Gain/1
  Acc/1(acc output) -> acc/1
  International Geomagnetic Reference Field/10 -> Terminator8/1
  Constant1/1 -> International Geomagnetic Reference Field/2
  International Geomagnetic Reference Field/6 -> Terminator3/1
  Sum/1 -> Mag/1(real mag data)  "real mag"
  Vel Imu/1(acc output) -> velocity IMU/1
  International Geomagnetic Reference Field/4 -> Terminator2/1
  Mag/1(mag output) -> Degrees to Radians/1
  International Geomagnetic Reference Field/1 -> Terminator/1
  Gain/1 -> Sum/2
  International Geomagnetic Reference Field/2 -> Terminator1/1
  gyro/1(Gyro output) -> "gyro "/1
  Constant3/1 -> International Geomagnetic Reference Field/4
  Transport Delay3/1 -> Acc/1(real acc data)
  Transport Delay/1 -> Quaternions to Rotation Angles/1

== system Aearial_Inspection_UAV_Simulation/GPS-INS/demux ==
  Sensors : Inport
  Acceleration Composer : Mux  Inputs=3
  Angular Velocity Composer : Mux  Inputs=3
  Demux : Demux  Outputs=9+4+3+3
  Position Composer : Mux  Inputs=3
  Quaternion Composer : Mux
  Terminator : Terminator
  Terminator1 : Terminator
  Terminator2 : Terminator
  Velocity Composer : Mux  Inputs=3
  Angular Velocity : Outport
  Quaternion : Outport  Port=2
  Acceleration : Outport  Port=3
  Velocity : Outport  Port=4
  Position : Outport  Port=5
  wires:
  Demux/13 -> Quaternion Composer/4
  Demux/3 -> Acceleration Composer/1
  Demux/14 -> Angular Velocity Composer/1
  Demux/5 -> Velocity Composer/2
  Demux/6 -> Acceleration Composer/2
  Demux/2 -> Velocity Composer/1
  Demux/16 -> Angular Velocity Composer/3
  Demux/9 -> Acceleration Composer/3
  Demux/4 -> Position Composer/2
  Demux/1 -> Position Composer/1
  Demux/18 -> Terminator1/1
  Demux/7 -> Position Composer/3
  Demux/15 -> Angular Velocity Composer/2
  Quaternion Composer/1 -> Quaternion/1
  Demux/8 -> Velocity Composer/3
  Demux/17 -> Terminator/1
  Sensors/1 -> Demux/1
  Position Composer/1 -> Position/1
  Angular Velocity Composer/1 -> Angular Velocity/1
  Demux/10 -> Quaternion Composer/1
  Demux/19 -> Terminator2/1
  Velocity Composer/1 -> Velocity/1
  Demux/11 -> Quaternion Composer/2
  Demux/12 -> Quaternion Composer/3
  Acceleration Composer/1 -> Acceleration/1

== system Aearial_Inspection_UAV_Simulation/Path Palnner/Arm Guid ==
  Mode : Inport
  ArmMode : Inport  Port=2
  uav_pos : Inport  Port=3
  Guidance Gate : Subsystem
      settings: PortSchema="{\"entries\":[{\"content\":{\"sides\":[{\"content\":{\"connectorIds\":[\"In1\",\"In2\"]},\"type\":\"ConnectorPlacement.EquallySpacedRectSide\",\"uuid\":\"b584fbf4-3ec9-4aac-9723-f8fdb4d6b5d3\"},{\"content\":{\"connectorIds\":[\"Out1\",\"Out2\"],\"side\":\"RIGHT\"},\"type\":\"ConnectorPlacement.EquallySpacedRectSide\",\"uuid\":\"d63ea83a-c528-47c2-b82a-c47989a7bba7\"},{\"content\":{\"connectorIds\":[\"In3\",\"In4\",\"In5\",\"In6\",\"In7\",\"In8\"],\"side\":\"TOP\"},\"type\":\"ConnectorPlacement.EquallySpacedRectSide\",\"uuid\":\"cea15c43-45f3-40c8-bad3-f304f0dbfb65\"},{\"content\":{\"connectorIds\":[\"In9\",\"In10\",\"In11\",\"In12\"],\"side\":\"BOTTOM\"},\"type\":\"ConnectorPlacement.EquallySpacedRectSide\",\"uuid\":\"8b3282b7-277b-4ce3-a51e-9f7c29937239\"}]},\"type\":\"ConnectorPlacement.EquallySpacedConnector\",\"uuid\":\"9e559c16-7068-490c-a42c-6800405b69e7\"}],\"packageUris\":[\"http://schema.mathworks.com/mf0/Connector/R2020b\"],\"version\":\"1.0\"}"
      mask Display: disp("Gate")
  Manual : Subsystem  Commented=on
  Senario 1 : Subsystem
  Senario 2 : Subsystem
  Senario 3 : Subsystem
  Senario 4 : Subsystem
  Senario 5 : Subsystem
  if Mode == Manual : simulink/Logic and Bit Operations/Compare To Constant  relop===  const=0  OutDataTypeStr=boolean
  if Mode == Senario 1 : simulink/Logic and Bit Operations/Compare To Constant  relop===  const=1  OutDataTypeStr=boolean
  if Mode == Senario 2 : simulink/Logic and Bit Operations/Compare To Constant  relop===  const=2  OutDataTypeStr=boolean
  if Mode == Senario 3 : simulink/Logic and Bit Operations/Compare To Constant  relop===  const=3  OutDataTypeStr=boolean
  if Mode == Senario 4 : simulink/Logic and Bit Operations/Compare To Constant  relop===  const=4  OutDataTypeStr=boolean
  if Mode == Senario 5 : simulink/Logic and Bit Operations/Compare To Constant  relop===  const=5  OutDataTypeStr=boolean
  Arm_desired_pos : Outport
  Arm Desired Orientation : Outport  Port=2
  wires:
  Senario 2/1(desired position) -> Guidance Gate/9(pos Sen 2)
  if Mode == Manual/1 -> Manual/Enable
  Manual/1(desired position) -> Guidance Gate/4(Manual pos)
  if Mode == Senario 2/1 -> Senario 2/Enable
  Senario 5/2(desired Heading) -> Guidance Gate/7(psi sen 5)
  Guidance Gate/2(desired Heading) -> Arm Desired Orientation/1  "Arm Desired Orientation"
  Senario 4/1(desired position) -> Guidance Gate/6(pos Sen 4)
  Senario 3/2(desired Heading) -> Guidance Gate/12(psi sen 3)
  Senario 4/2(desired Heading) -> Guidance Gate/5(psi sen 4)
  Guidance Gate/1(desired position) -> Arm_desired_pos/1  "Arm_desired_pos"
  Senario 1/2(desired Heading) -> Guidance Gate/2(psi sen 1)
  Senario 1/1(desired position) -> Guidance Gate/1(Sen1 pos)
  Manual/2(desired Heading) -> Guidance Gate/3(Manual psi)
  Mode/1 -> if Mode == Senario 3/1, if Mode == Senario 2/1, if Mode == Senario 5/1, if Mode == Senario 4/1, if Mode == Manual/1, if Mode == Senario 1/1
  Senario 5/1(desired position) -> Guidance Gate/8(pos Sen 5)
  if Mode == Senario 5/1 -> Senario 5/Enable
  Senario 2/2(desired Heading) -> Guidance Gate/10(psi sen 2)
  if Mode == Senario 3/1 -> Senario 3/Enable
  if Mode == Senario 4/1 -> Senario 4/Enable
  Senario 3/1(desired position) -> Guidance Gate/11(pos Sen 3)
  if Mode == Senario 1/1 -> Senario 1/Enable
  ArmMode/1 -> Senario 5/1(ArmMode)
  uav_pos/1 -> Senario 5/2(uav_pos)

== system Aearial_Inspection_UAV_Simulation/Path Palnner/UAV_Guid ==
  Mode : Inport
  Guidance Gate : Subsystem
      settings: PortSchema="{\"entries\":[{\"content\":{\"sides\":[{\"content\":{\"connectorIds\":[\"In1\",\"In2\"]},\"type\":\"ConnectorPlacement.EquallySpacedRectSide\",\"uuid\":\"b584fbf4-3ec9-4aac-9723-f8fdb4d6b5d3\"},{\"content\":{\"connectorIds\":[\"Out1\",\"Out2\"],\"side\":\"RIGHT\"},\"type\":\"ConnectorPlacement.EquallySpacedRectSide\",\"uuid\":\"d63ea83a-c528-47c2-b82a-c47989a7bba7\"},{\"content\":{\"connectorIds\":[\"In3\",\"In4\",\"In5\",\"In6\",\"In7\",\"In8\"],\"side\":\"TOP\"},\"type\":\"ConnectorPlacement.EquallySpacedRectSide\",\"uuid\":\"cea15c43-45f3-40c8-bad3-f304f0dbfb65\"},{\"content\":{\"connectorIds\":[\"In9\",\"In10\",\"In11\",\"In12\"],\"side\":\"BOTTOM\"},\"type\":\"ConnectorPlacement.EquallySpacedRectSide\",\"uuid\":\"8b3282b7-277b-4ce3-a51e-9f7c29937239\"}]},\"type\":\"ConnectorPlacement.EquallySpacedConnector\",\"uuid\":\"9e559c16-7068-490c-a42c-6800405b69e7\"}],\"packageUris\":[\"http://schema.mathworks.com/mf0/Connector/R2020b\"],\"version\":\"1.0\"}"
      mask Display: disp("Gate")
  Manual : Subsystem  Commented=on
  Senario 1 : Subsystem
  Senario 2 : Subsystem
  Senario 3 : Subsystem
  Senario 4 : Subsystem
  Senario 5 : Subsystem
  angle jump correction : Subsystem
  if Mode == Manual : simulink/Logic and Bit Operations/Compare To Constant  relop===  const=0  OutDataTypeStr=boolean
  if Mode == Manual1 : simulink/Logic and Bit Operations/Compare To Constant  relop===  const=4  OutDataTypeStr=boolean
  if Mode == Manual2 : simulink/Logic and Bit Operations/Compare To Constant  relop===  const=5  OutDataTypeStr=boolean
  if Mode == Senario 1 : simulink/Logic and Bit Operations/Compare To Constant  relop===  const=1  OutDataTypeStr=boolean
  if Mode == Senario 2 : simulink/Logic and Bit Operations/Compare To Constant  relop===  const=2  OutDataTypeStr=boolean
  if Mode == Senario 3 : simulink/Logic and Bit Operations/Compare To Constant  relop===  const=3  OutDataTypeStr=boolean
  desired_pos : Outport
  desired Heading : Outport  Port=2
  wires:
  if Mode == Manual/1 -> Manual/Enable
  Senario 1/1(desired position) -> Guidance Gate/1(Sen1 pos)
  if Mode == Senario 2/1 -> Senario 2/Enable
  Manual/1(desired position) -> Guidance Gate/4(Manual pos)
  Senario 1/2(desired Heading) -> Guidance Gate/2(psi sen 1)
  Senario 2/1(desired position) -> Guidance Gate/9(pos Sen 2)
  Senario 3/2(desired Heading) -> Guidance Gate/12(psi sen 3)
  Senario 3/1(desired position) -> Guidance Gate/11(pos Sen 3)
  Senario 2/2(desired Heading) -> Guidance Gate/10(psi sen 2)
  Senario 5/1(desired position) -> Guidance Gate/8(pos Sen 5)
  if Mode == Senario 3/1 -> Senario 3/Enable
  Guidance Gate/1(desired position) -> desired_pos/1  "desired pos"
  Manual/2(desired Heading) -> Guidance Gate/3(Manual psi)
  Senario 5/2(desired Heading) -> Guidance Gate/7(psi sen 5)
  Mode/1 -> if Mode == Senario 3/1, if Mode == Senario 2/1, if Mode == Manual2/1, if Mode == Manual1/1, if Mode == Manual/1, if Mode == Senario 1/1
  if Mode == Manual1/1 -> Senario 4/Enable
  if Mode == Manual2/1 -> Senario 5/Enable
  Guidance Gate/2(desired Heading) -> angle jump correction/1(u)  "desired Heading"
  Senario 4/1(desired position) -> Guidance Gate/6(pos Sen 4)
  Senario 4/2(desired Heading) -> Guidance Gate/5(psi sen 4)
  if Mode == Senario 1/1 -> Senario 1/Enable
  angle jump correction/1(y) -> desired Heading/1

== system Aearial_Inspection_UAV_Simulation/UAV/Camera ==
  tilt_angle : Inport
  Roll_angle : Inport  Port=2
  Camera_Gripper_1_2_RIGID : Subsystem
  Constant : Constant  Value=180
  FPV_Camera_1_RIGID : Subsystem
  Integrator{1..2,6..7} (4 alike) : Integrator
  Mux : Mux  Inputs=2
  Revolute13 : sm_lib/Joints/Revolute Joint  JointMode=Normal  SenseConstraintForce=off  SenseConstraintForceX=off  SenseConstraintForceY=off  SenseConstraintForceZ=off  SenseConstraintTorque=off  SenseConstraintTorqueX=off  SenseConstraintTorqueY=off  SenseConstraintTorqueZ=off  SenseTotalForce=off  SenseTotalForceX=off  SenseTotalForceY=off  SenseTotalForceZ=off  SenseTotalTorque=off  SenseTotalTorqueX=off  SenseTotalTorqueY=off  SenseTotalTorqueZ=off  CompositeWrenchDir=FollowerOnBase  CompositeWrenchFrame=BaseFrame  EquilibriumPosition=0  EquilibriumPositionUnits=deg  SpringStiffness=0  SpringStiffnessUnits=N*m/deg  DampingCoefficient=0  DampingCoefficientUnits=N*m/(deg/s)  TorqueActuationMode=ComputedTorque  MotionActuationMode=InputMotion  SensePosition=off  SenseVelocity=off  SenseAcceleration=off  SenseTorqueForce=off  SenseLowerLimitTorqueForce=off  SenseUpperLimitTorqueForce=off  LowerLimitSpecify=off  LowerLimitBound=-90  LowerLimitBoundUnits=deg  LowerLimitStiffness=1e4  LowerLimitStiffnessUnits=N*m/deg  LowerLimitDamping=10  LowerLimitDampingUnits=N*m/(deg/s)  LowerLimitTransitionRegionWidth=0.1  LowerLimitTransitionRegionWidthUnits=deg  UpperLimitSpecify=off  UpperLimitBound=90  UpperLimitBoundUnits=deg  UpperLimitStiffness=1e4  UpperLimitStiffnessUnits=N*m/deg  UpperLimitDamping=10  UpperLimitDampingUnits=N*m/(deg/s)  UpperLimitTransitionRegionWidth=0.1  UpperLimitTransitionRegionWidthUnits=deg  PositionTargetSpecify=on  PositionTargetPriority=Low  PositionTargetValue=smiData.RevoluteJoint(14).Rz.Pos  PositionTargetValueUnits=deg  VelocityTargetSpecify=off  VelocityTargetPriority=High  VelocityTargetValue=0  VelocityTargetValueUnits=deg/s
  Revolute15 : sm_lib/Joints/Revolute Joint  JointMode=Normal  SenseConstraintForce=off  SenseConstraintForceX=off  SenseConstraintForceY=off  SenseConstraintForceZ=off  SenseConstraintTorque=off  SenseConstraintTorqueX=off  SenseConstraintTorqueY=off  SenseConstraintTorqueZ=off  SenseTotalForce=off  SenseTotalForceX=off  SenseTotalForceY=off  SenseTotalForceZ=off  SenseTotalTorque=off  SenseTotalTorqueX=off  SenseTotalTorqueY=off  SenseTotalTorqueZ=off  CompositeWrenchDir=FollowerOnBase  CompositeWrenchFrame=BaseFrame  EquilibriumPosition=0  EquilibriumPositionUnits=deg  SpringStiffness=0  SpringStiffnessUnits=N*m/deg  DampingCoefficient=0  DampingCoefficientUnits=N*m/(deg/s)  TorqueActuationMode=ComputedTorque  MotionActuationMode=InputMotion  SensePosition=off  SenseVelocity=off  SenseAcceleration=off  SenseTorqueForce=off  SenseLowerLimitTorqueForce=off  SenseUpperLimitTorqueForce=off  LowerLimitSpecify=off  LowerLimitBound=-90  LowerLimitBoundUnits=deg  LowerLimitStiffness=1e4  LowerLimitStiffnessUnits=N*m/deg  LowerLimitDamping=10  LowerLimitDampingUnits=N*m/(deg/s)  LowerLimitTransitionRegionWidth=0.1  LowerLimitTransitionRegionWidthUnits=deg  UpperLimitSpecify=off  UpperLimitBound=90  UpperLimitBoundUnits=deg  UpperLimitStiffness=1e4  UpperLimitStiffnessUnits=N*m/deg  UpperLimitDamping=10  UpperLimitDampingUnits=N*m/(deg/s)  UpperLimitTransitionRegionWidth=0.1  UpperLimitTransitionRegionWidthUnits=deg  PositionTargetSpecify=on  PositionTargetPriority=Low  PositionTargetValue=smiData.RevoluteJoint(16).Rz.Pos  PositionTargetValueUnits=deg  VelocityTargetSpecify=off  VelocityTargetPriority=High  VelocityTargetValue=0  VelocityTargetValueUnits=deg/s
  Simulink-PS Converter1 : nesl_utility/Simulink-PS Converter  PhysicalDomain=network_engine_domain  SubClassName=ps_input  LeftPortType=input  RightPortType=output  PseudoPeriodic=off  Frequencies=[]  NoiseDistribution=none  NoiseParameters=[]  Unit=deg  AffineConversion=off  FilteringAndDerivatives=provide  SimscapeFilterOrder=1  InputFilterTimeConstant=0.001  UdotUserProvided=2
  Simulink-PS Converter3 : nesl_utility/Simulink-PS Converter  PhysicalDomain=network_engine_domain  SubClassName=ps_input  LeftPortType=input  RightPortType=output  PseudoPeriodic=off  Frequencies=[]  NoiseDistribution=none  NoiseParameters=[]  Unit=deg  AffineConversion=off  FilteringAndDerivatives=provide  SimscapeFilterOrder=1  InputFilterTimeConstant=0.001  UdotUserProvided=2
  Sum : Sum  Inputs=++|
  Transfer Fcn1 : TransferFcn  Numerator=[stepper.wn^2 0 0]  Denominator=[1 2*stepper.wn*stepper.zeta stepper.wn^2]
  Transfer Fcn2 : TransferFcn  Numerator=[stepper.wn^2 0 0]  Denominator=[1 2*stepper.wn*stepper.zeta stepper.wn^2]
  Arm : PMIOPort  Side=Left
  Camera rotation [Roll Tilt] [deg] : Outport
  wires:
  Transfer Fcn2/1 -> Simulink-PS Converter3/3, Integrator6/1
  Integrator6/1 -> Simulink-PS Converter3/2, Integrator7/1
  tilt_angle/1 -> Transfer Fcn2/1
  Integrator7/1 -> Mux/2, Simulink-PS Converter3/1
  Roll_angle/1 -> Transfer Fcn1/1
  Integrator1/1 -> Simulink-PS Converter1/2, Integrator2/1
  Transfer Fcn1/1 -> Simulink-PS Converter1/3, Integrator1/1
  Integrator2/1 -> Mux/1, Sum/2
  Sum/1 -> Simulink-PS Converter1/1
  Constant/1 -> Sum/1
  Mux/1 -> Camera rotation [Roll Tilt] [deg]/1
  connections:
  Camera_Gripper_1_2_RIGID/LConn2 -- Revolute13/RConn1
  Arm/RConn1 -- Revolute13/LConn1
  Camera_Gripper_1_2_RIGID/LConn1 -- Revolute15/RConn1
  Revolute15/LConn1 -- FPV_Camera_1_RIGID/RConn1
  Simulink-PS Converter3/RConn1 -- Revolute15/LConn2
  Simulink-PS Converter1/RConn1 -- Revolute13/LConn2
